simulink model "model_notlin"  (R2020b)
settings: Solver=ode45  StartTime=0.0  StopTime=10  MaxStep=0.01  RelTol=1e-3
undefined symbols (not defined in the file): params
settings Model: Creator=Danil  LastModifiedBy=Danil

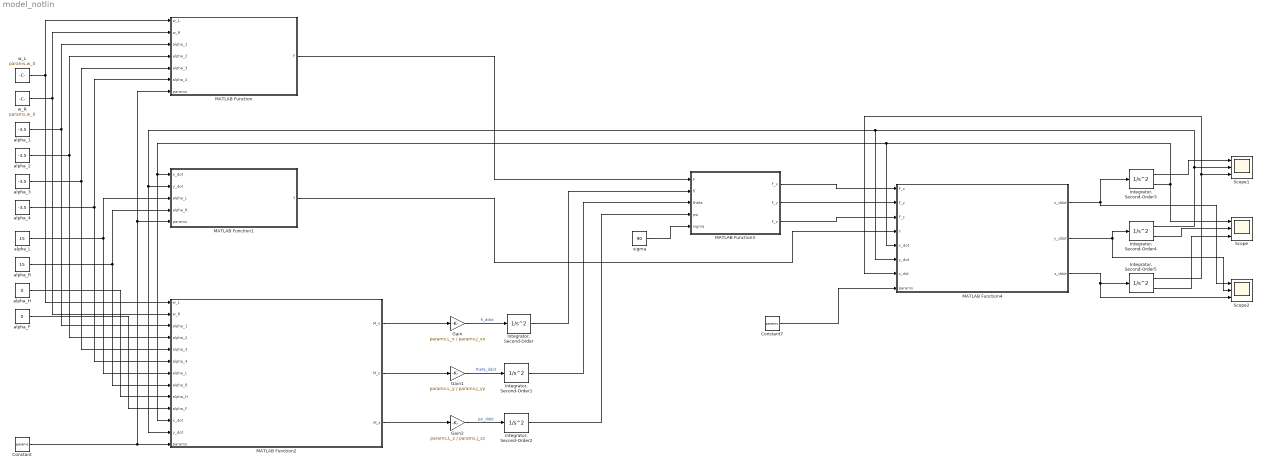
== system model_notlin ==
  Constant : Constant  Value=params  OutDataTypeStr=Bus: params_bus
  Constant7 : Constant  Value=params  OutDataTypeStr=Bus: params_bus
  Gain : Gain  Gain=params.L_x / params.J_xx
  Gain1 : Gain  Gain=params.L_y / params.J_yy
  Gain2 : Gain  Gain=params.L_z / params.J_zz
  "Integrator, Second-Order" : SecondOrderIntegrator  ShowOutput=x
  "Integrator, Second-Order1" : SecondOrderIntegrator  ShowOutput=x
  "Integrator, Second-Order2" : SecondOrderIntegrator  ShowOutput=x
  "Integrator, Second-Order3" : SecondOrderIntegrator
  "Integrator, Second-Order4" : SecondOrderIntegrator
  "Integrator, Second-Order5" : SecondOrderIntegrator
  MATLAB Function : MATLAB Function  TreatAsAtomicUnit=on
  MATLAB Function1 : MATLAB Function  TreatAsAtomicUnit=on
  MATLAB Function2 : MATLAB Function  TreatAsAtomicUnit=on
  MATLAB Function3 : MATLAB Function  TreatAsAtomicUnit=on
  MATLAB Function4 : MATLAB Function  TreatAsAtomicUnit=on
  Scope : Scope  NumInputPorts=3
  Scope1 : Scope  NumInputPorts=3
  Scope2 : Scope  NumInputPorts=3
  alpha_{1..4} (4 alike) : Constant  Value=-3.5
  alpha_F : Constant  Value=0
  alpha_H : Constant  Value=0
  alpha_L : Constant  Value=15
  alpha_R : Constant  Value=15
  sigma : Constant  Value=90
  w_L : Constant  Value=params.w_0
  w_R : Constant  Value=params.w_0
  wires:
  Gain/1 -> "Integrator, Second-Order"/1  "fi_ddot"
  Gain1/1 -> "Integrator, Second-Order1"/1  "theta_ddot"
  Gain2/1 -> "Integrator, Second-Order2"/1  "psi_ddot"
  MATLAB Function4/1(x_ddot) -> "Integrator, Second-Order3"/1, Scope2/1
  MATLAB Function4/2(y_ddot) -> "Integrator, Second-Order4"/1, Scope2/2
  MATLAB Function4/3(z_ddot) -> Scope2/3, "Integrator, Second-Order5"/1
  "Integrator, Second-Order3"/2 -> Scope/1, MATLAB Function2/11(x_dot), MATLAB Function1/1(x_dot), MATLAB Function4/5(x_dot)
  "Integrator, Second-Order4"/2 -> Scope/2
  "Integrator, Second-Order5"/2 -> Scope/3
  "Integrator, Second-Order3"/1 -> Scope1/1
  "Integrator, Second-Order4"/1 -> MATLAB Function2/12(y_dot), MATLAB Function1/2(y_dot), MATLAB Function4/6(y_dot), Scope1/2
  "Integrator, Second-Order5"/1 -> Scope1/3, MATLAB Function4/7(z_dot)
  MATLAB Function3/2(F_y) -> MATLAB Function4/2(F_y)
  MATLAB Function3/1(F_x) -> MATLAB Function4/1(F_x)
  MATLAB Function3/3(F_z) -> MATLAB Function4/3(F_z)
  Constant7/1 -> MATLAB Function4/8(params)
  w_L/1 -> MATLAB Function/1(w_L), MATLAB Function2/1(w_L)
  w_R/1 -> MATLAB Function/2(w_R), MATLAB Function2/2(w_R)
  alpha_1/1 -> MATLAB Function/3(alpha_1), MATLAB Function2/3(alpha_1)
  alpha_2/1 -> MATLAB Function/4(alpha_2), MATLAB Function2/4(alpha_2)
  alpha_3/1 -> MATLAB Function/5(alpha_3), MATLAB Function2/5(alpha_3)
  alpha_4/1 -> MATLAB Function/6(alpha_4), MATLAB Function2/6(alpha_4)
  Constant/1 -> MATLAB Function2/13(params), MATLAB Function1/5(params), MATLAB Function/7(params)
  alpha_L/1 -> MATLAB Function1/3(alpha_L), MATLAB Function2/7(alpha_L)
  alpha_R/1 -> MATLAB Function1/4(alpha_R), MATLAB Function2/8(alpha_R)
  alpha_H/1 -> MATLAB Function2/9(alpha_H)
  alpha_F/1 -> MATLAB Function2/10(alpha_F)
  MATLAB Function2/1(M_x) -> Gain/1
  MATLAB Function2/2(M_y) -> Gain1/1
  MATLAB Function2/3(M_z) -> Gain2/1
  MATLAB Function/1(F) -> MATLAB Function3/1(F)
  MATLAB Function1/1(Y) -> MATLAB Function4/4(Y)
  "Integrator, Second-Order"/1 -> MATLAB Function3/2(fi)
  "Integrator, Second-Order1"/1 -> MATLAB Function3/3(theta)
  "Integrator, Second-Order2"/1 -> MATLAB Function3/4(psi)
  sigma/1 -> MATLAB Function3/5(sigma)

== matlab function model_notlin/MATLAB Function1 ==
  data: x_dot input; y_dot input; alpha_L input; alpha_R input; params input; Y output
function Y = fcn(x_dot, y_dot, alpha_L, alpha_R, params)

C_y_L = params.a_k * alpha_L^2 + params.b_k * alpha_L + params.c_k;
C_y_R = params.a_k * alpha_R^2 + params.b_k * alpha_R + params.c_k;

Y = (1 / 2) * params.rho * (x_dot^2 + y_dot^2) * params.S_k * (C_y_L + C_y_R);

== matlab function model_notlin/MATLAB Function ==
  data: w_L input; F output; w_R input; alpha_1 input; alpha_2 input; alpha_3 input; alpha_4 input; params input
function F  = fcn(w_L, w_R, alpha_1, alpha_2, alpha_3, alpha_4, params)

alpha_L = alpha_1 + alpha_2;
alpha_R = alpha_3 + alpha_4;

C_Y_L = params.a_l * alpha_L^2 + params.b_l * alpha_L + params.c_l;
C_Y_R = params.a_l * alpha_R^2 + params.b_l * alpha_R + params.c_l;

F = (3/2) * params.rho * params.S_l * (C_Y_L * w_L^2 + C_Y_R * w_R^2);

== matlab function model_notlin/MATLAB Function2 ==
  data: w_L input; w_R input; alpha_1 input; alpha_2 input; alpha_3 input; alpha_4 input; alpha_L input; alpha_R input; alpha_H input; alpha_F input; x_dot input; y_dot input; M_x output; M_y output; M_z output; params input
function [M_x, M_y, M_z] = fcn(w_L, w_R, alpha_1, alpha_2, alpha_3, alpha_4, ...
                               alpha_L, alpha_R, alpha_H, alpha_F, x_dot, y_dot, params)

C_y_L_l_x = params.a_l * (alpha_1 + alpha_2)^2 + params.b_l * (alpha_1 + alpha_2) + params.c_l;
C_y_R_l_x = params.a_l * (alpha_3 + alpha_4)^2 + params.b_l * (alpha_3 + alpha_4) + params.c_l;

C_y_L_l_yz = params.a_l * (alpha_1 - alpha_2)^2 + params.b_l * (alpha_1 - alpha_2) + params.c_l;
C_y_R_l_yz = params.a_l * (alpha_3 - alpha_4)^2 + params.b_l * (alpha_3 - alpha_4) + params.c_l;

C_y_L_k = params.a_k * alpha_L^2 + params.b_k * alpha_L + params.c_k;
C_y_R_k = params.a_k * alpha_R^2 + params.b_k * alpha_R + params.c_k;

C_y_H = params.a_h * alpha_H^3 + params.b_h * alpha_H^2 + params.c_h * alpha_H + params.d_h;
C_y_F = params.a_f * alpha_F^3 + params.b_f * alpha_F^2 + params.c_f * alpha_F + params.d_f;

M_x = ((3 / 2) * params.rho * params.S_l * (C_y_L_l_x * w_L^2 - C_y_R_l_x * w_R^2)) + ...
      ((1 / 2) * params.rho * params.S_k * (x_dot^2 + y_dot^2) * (C_y_L_k - C_y_R_k));
  
M_y = ((3 / 2) * params.rho * params.S_l * (C_y_L_l_yz * w_L^2 + C_y_R_l_yz * w_R^2)) + ...
      ((1 / 2) * C_y_H * params.rho * params.S_h * (x_dot^2 + y_dot^2));
  
M_z = ((3 / 2) * params.rho * params.S_l * (C_y_L_l_yz * w_L^2 - C_y_R_l_yz * w_R^2)) + ...
      ((1 / 2) * C_y_F * params.rho * params.S_f * (x_dot^2 + y_dot^2));

== matlab function model_notlin/MATLAB Function3 ==
  data: F input; F_x output; fi input; theta input; psi input; F_y output; F_z output; sigma input
function [F_x, F_y, F_z] = fcn(F, fi, theta, psi, sigma)

sigma = sigma * pi / 180;

F_x = F * sin(sigma) * (cos(psi) * sin(theta) + cos(theta) * sin(fi) * sin(psi)) + F * cos(sigma) * (cos(psi) * cos(theta));
F_y = F * sin(sigma) * (sin(psi) * sin(theta) - cos(psi) * cos(theta) * sin(fi)) + F * cos(sigma) * (cos(fi) * sin(psi) + cos(psi) * sin(fi) * sin(theta));
F_z = F * sin(sigma) * (cos(fi) * cos(theta)) + F * cos(sigma) * (sin(fi) * sin(psi) - cos(fi) * cos(psi) * sin(theta));

== matlab function model_notlin/MATLAB Function4 ==
  data: F_x input; x_ddot output; F_y input; F_z input; Y input; x_dot input; y_dot input; z_dot input; params input; y_ddot output; z_ddot output
function [x_ddot, y_ddot, z_ddot] = fcn(F_x, F_y, F_z, Y, x_dot, y_dot, z_dot, params)

x_ddot = (1 / params.m) * (F_x - params.k_x * x_dot);
y_ddot = (1 / params.m) * (F_y - params.k_y * y_dot);
z_ddot = (1 / params.m) * (F_z + Y - params.k_z * z_dot - params.m * params.g);
